simulink model "TEST"  (R2021a)
settings: Solver=VariableStepAuto  StartTime=0.0  StopTime=50  FixedStep=0.001  RelTol=1e-3
values from neighbouring files (symbols this model uses):
  B = inv(N)    [Para.m]    (also in Parameters.m = inv(N)*[zeros(3);eye(3)])
  dtheta_LMO = sqrt(muy/r_LMO^3)    [Para.m]    (also in Parameters.m)
  i0_LMO = pi/6    (= 0.523598775598)    [Para.m]    (also in Parameters.m)
  N = [eye(3) zeros(3);zeros(3) J]    [Dynamics.m]    (also in Para.m; Parameters.m)
  Omega0_LMO = pi/9    (= 0.349065850399)    [Para.m]    (also in Parameters.m)
  R = eye(6)    [Para.m]    (also in Parameters.m = eye(3))
  S = [0 0 0 0.5 0 0;           0 0 0 0 0.5 0;           0 0 0 0 0 0.5;           f41 0 0 0 0 f46;           0 f52 0 0 0 0;           0 0 f63 f64 0 0]    [Para.m]    (also in Parameters.m; crossMatrix.m = [0 -q3 q2;           q3 0 -q1;           -q2 q1 0])
  theta0_LMO = pi/3    (= 1.0471975512)    [Para.m]    (also in Parameters.m)
undefined symbols (not defined in the file or in its folder): F
libraries: dspsrcs4 x1
settings Model: Creator=VTX  LastModifiedBy=VTX

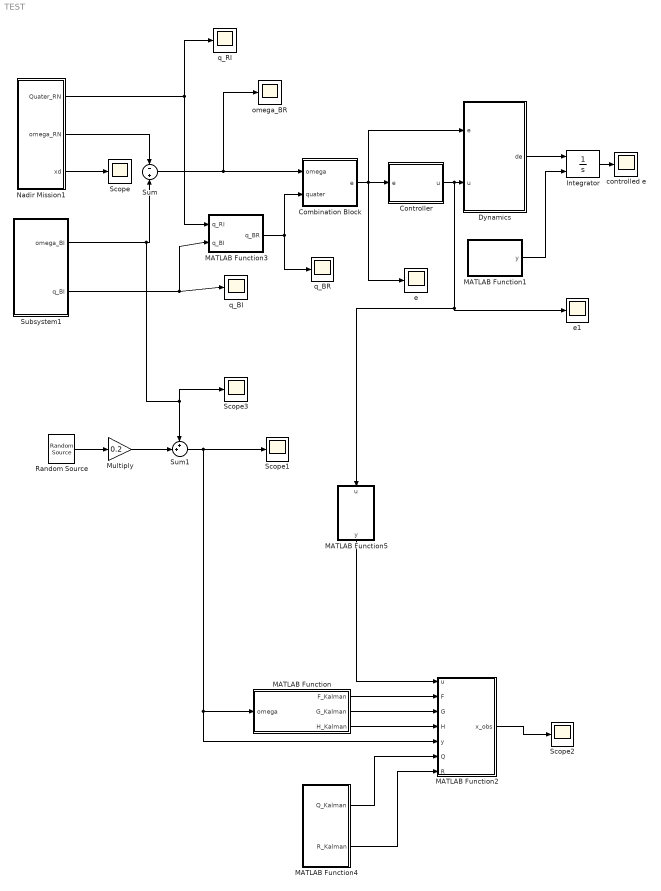
== system TEST ==
  Combination Block : Subsystem
  Controller : MATLAB Function  TreatAsAtomicUnit=on
  Dynamics : MATLAB Function  TreatAsAtomicUnit=on
  Integrator : Integrator  InitialConditionSource=external
  MATLAB Function : MATLAB Function  TreatAsAtomicUnit=on
  MATLAB Function1 : MATLAB Function  TreatAsAtomicUnit=on
  MATLAB Function2 : MATLAB Function  TreatAsAtomicUnit=on
  MATLAB Function3 : MATLAB Function  TreatAsAtomicUnit=on
  MATLAB Function4 : MATLAB Function  TreatAsAtomicUnit=on
  MATLAB Function5 : MATLAB Function  TreatAsAtomicUnit=on
  Multiply : Gain  Gain=0.2
  Nadir Mission1 : Subsystem
  Random Source : dspsrcs4/Random Source  SrcType=Uniform  NormMethod=Ziggurat  CltLength=12  MinVal=0  MaxVal=1  MeanVal=0  VarVal=1  RepMode=Not repeatable  rawSeed=1  IsInherit=off  SampMode=Discrete  SampTime=0.05  SampFrame=1  DataType=Double  OutComplex=Real  OutputFrames=off
  Scope{,1..3} (4 alike) : Scope
  Subsystem1 : Subsystem
  Sum : Sum  Inputs=-|+
  Sum1 : Sum  Inputs=++|
  controlled e : Scope
  e : Scope
  e1 : Scope
  omega_BR : Scope
  q_BI : Scope
  q_BR : Scope
  q_RI : Scope
  wires:
  Controller/1(u) -> MATLAB Function5/1(u), e1/1, Dynamics/2(u)
  Integrator/1 -> controlled e/1
  Dynamics/1(de) -> Integrator/1
  Nadir Mission1/2(omega_RN) -> Sum/1
  Nadir Mission1/3(xd) -> Scope/1
  Nadir Mission1/1(Quater_RN) -> q_RI/1, MATLAB Function3/1(q_RI)
  MATLAB Function3/1(q_BR) -> Combination Block/2(quater), q_BR/1
  Combination Block/1(e) -> e/1, Dynamics/1(e), Controller/1(e)
  Sum/1 -> Combination Block/1(omega), omega_BR/1
  MATLAB Function1/1(y) -> Integrator/2
  Subsystem1/1(omega_BI) -> Scope3/1, Sum1/1, Sum/2
  Subsystem1/2(q_BI) -> q_BI/1, MATLAB Function3/2(q_BI)
  Sum1/1 -> MATLAB Function2/5(y), MATLAB Function/1(omega), Scope1/1
  Random Source/1 -> Multiply/1
  Multiply/1 -> Sum1/2
  MATLAB Function/1(F_Kalman) -> MATLAB Function2/2(F)
  MATLAB Function/2(G_Kalman) -> MATLAB Function2/3(G)
  MATLAB Function/3(H_Kalman) -> MATLAB Function2/4(H)
  MATLAB Function4/1(Q_Kalman) -> MATLAB Function2/6(Q)
  MATLAB Function4/2(R_Kalman) -> MATLAB Function2/7(R)
  MATLAB Function2/1(x_obs) -> Scope2/1
  MATLAB Function5/1(y) -> MATLAB Function2/1(u)

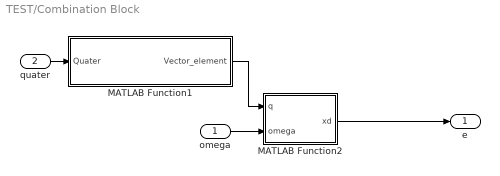
== system TEST/Combination Block ==
  omega : Inport
  quater : Inport  Port=2
  MATLAB Function1 : MATLAB Function  TreatAsAtomicUnit=on
  MATLAB Function2 : MATLAB Function  TreatAsAtomicUnit=on
  e : Outport
  wires:
  MATLAB Function2/1(xd) -> e/1
  MATLAB Function1/1(Vector_element) -> MATLAB Function2/1(q)
  quater/1 -> MATLAB Function1/1(Quater)
  omega/1 -> MATLAB Function2/2(omega)

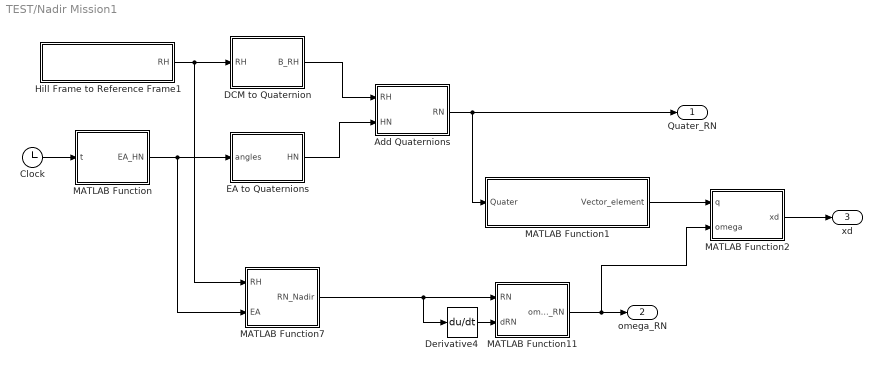
== system TEST/Nadir Mission1 ==
  Add Quaternions : MATLAB Function  TreatAsAtomicUnit=on
  Clock : Clock
  DCM to Quaternion : MATLAB Function  TreatAsAtomicUnit=on
  Derivative4 : Derivative
  EA to Quaternions : MATLAB Function  TreatAsAtomicUnit=on
  Hill Frame to Reference Frame1 : MATLAB Function  TreatAsAtomicUnit=on
  MATLAB Function : MATLAB Function  TreatAsAtomicUnit=on
  MATLAB Function1 : MATLAB Function  TreatAsAtomicUnit=on
  MATLAB Function11 : MATLAB Function  TreatAsAtomicUnit=on
  MATLAB Function2 : MATLAB Function  TreatAsAtomicUnit=on
  MATLAB Function7 : MATLAB Function  TreatAsAtomicUnit=on
  Quater_RN : Outport
  omega_RN : Outport  Port=2
  xd : Outport  Port=3
  wires:
  Hill Frame to Reference Frame1/1(RH) -> MATLAB Function7/1(RH), DCM to Quaternion/1(RH)
  MATLAB Function/1(EA_HN) -> MATLAB Function7/2(EA), EA to Quaternions/1(angles)
  Clock/1 -> MATLAB Function/1(t)
  DCM to Quaternion/1(B_RH) -> Add Quaternions/1(RH)
  EA to Quaternions/1(HN) -> Add Quaternions/2(HN)
  Add Quaternions/1(RN) -> MATLAB Function1/1(Quater), Quater_RN/1
  MATLAB Function7/1(RN_Nadir) -> Derivative4/1, MATLAB Function11/1(RN)
  Derivative4/1 -> MATLAB Function11/2(dRN)
  MATLAB Function11/1(omega_RN) -> MATLAB Function2/2(omega), omega_RN/1
  MATLAB Function1/1(Vector_element) -> MATLAB Function2/1(q)
  MATLAB Function2/1(xd) -> xd/1

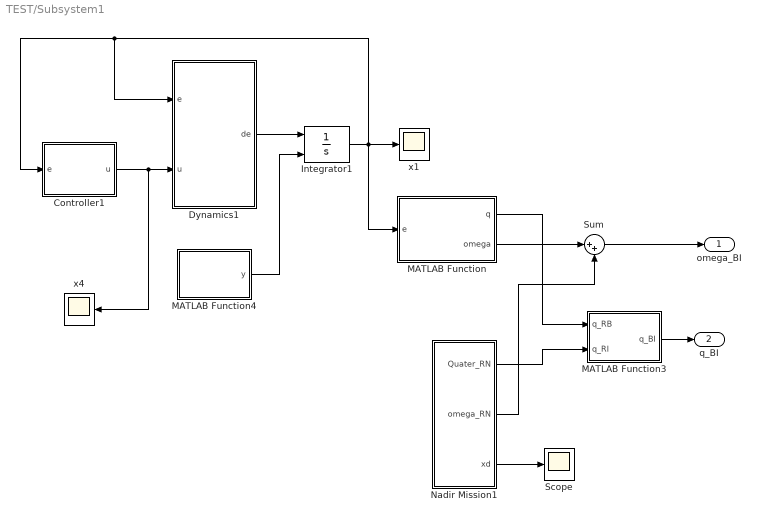
== system TEST/Subsystem1 ==
  Controller1 : MATLAB Function  TreatAsAtomicUnit=on
  Dynamics1 : MATLAB Function  TreatAsAtomicUnit=on
  Integrator1 : Integrator  InitialConditionSource=external
  MATLAB Function : MATLAB Function  TreatAsAtomicUnit=on
  MATLAB Function3 : MATLAB Function  TreatAsAtomicUnit=on
  MATLAB Function4 : MATLAB Function  TreatAsAtomicUnit=on
  Nadir Mission1 : Subsystem
  Scope : Scope
  Sum : Sum  Inputs=|++
  x1 : Scope
  x4 : Scope
  omega_BI : Outport
  q_BI : Outport  Port=2
  wires:
  Integrator1/1 -> MATLAB Function/1(e), Dynamics1/1(e), Controller1/1(e), x1/1
  Controller1/1(u) -> x4/1, Dynamics1/2(u)
  Dynamics1/1(de) -> Integrator1/1
  MATLAB Function4/1(y) -> Integrator1/2
  MATLAB Function/2(omega) -> Sum/1
  MATLAB Function/1(q) -> MATLAB Function3/1(q_RB)
  Nadir Mission1/1(Quater_RN) -> MATLAB Function3/2(q_RI)
  Nadir Mission1/2(omega_RN) -> Sum/2
  Nadir Mission1/3(xd) -> Scope/1
  Sum/1 -> omega_BI/1
  MATLAB Function3/1(q_BI) -> q_BI/1

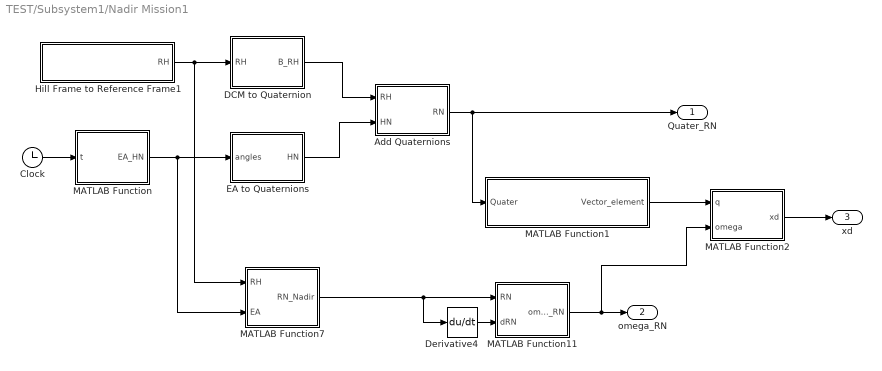
== system TEST/Subsystem1/Nadir Mission1 ==
  Add Quaternions : MATLAB Function  TreatAsAtomicUnit=on
  Clock : Clock
  DCM to Quaternion : MATLAB Function  TreatAsAtomicUnit=on
  Derivative4 : Derivative
  EA to Quaternions : MATLAB Function  TreatAsAtomicUnit=on
  Hill Frame to Reference Frame1 : MATLAB Function  TreatAsAtomicUnit=on
  MATLAB Function : MATLAB Function  TreatAsAtomicUnit=on
  MATLAB Function1 : MATLAB Function  TreatAsAtomicUnit=on
  MATLAB Function11 : MATLAB Function  TreatAsAtomicUnit=on
  MATLAB Function2 : MATLAB Function  TreatAsAtomicUnit=on
  MATLAB Function7 : MATLAB Function  TreatAsAtomicUnit=on
  Quater_RN : Outport
  omega_RN : Outport  Port=2
  xd : Outport  Port=3
  wires:
  Hill Frame to Reference Frame1/1(RH) -> MATLAB Function7/1(RH), DCM to Quaternion/1(RH)
  MATLAB Function/1(EA_HN) -> MATLAB Function7/2(EA), EA to Quaternions/1(angles)
  Clock/1 -> MATLAB Function/1(t)
  DCM to Quaternion/1(B_RH) -> Add Quaternions/1(RH)
  EA to Quaternions/1(HN) -> Add Quaternions/2(HN)
  Add Quaternions/1(RN) -> MATLAB Function1/1(Quater), Quater_RN/1
  MATLAB Function7/1(RN_Nadir) -> Derivative4/1, MATLAB Function11/1(RN)
  Derivative4/1 -> MATLAB Function11/2(dRN)
  MATLAB Function11/1(omega_RN) -> MATLAB Function2/2(omega), omega_RN/1
  MATLAB Function1/1(Vector_element) -> MATLAB Function2/1(q)
  MATLAB Function2/1(xd) -> xd/1

== matlab function TEST/Nadir Mission1/EA to Quaternions ==
  data: angles input; HN output
function HN = EulerAngles313_2_Quaternions(angles)
    Omega = angles(1);
    i = angles(2);
    omega = angles(3);

    q0 = cos(omega/2)*cos(i/2)*cos(Omega/2) - sin(omega/2)*cos(i/2)*sin(Omega/2);
    q1 = cos(omega/2)*sin(i/2)*cos(Omega/2) + sin(omega/2)*sin(i/2)*sin(Omega/2);
    q2 = -sin(omega/2)*sin(i/2)*cos(Omega/2) + cos(omega/2)*sin(i/2)*sin(Omega/2);
    q3 = sin(omega/2)*cos(i/2)*cos(Omega/2) + cos(omega/2)*cos(i/2)*sin(Omega/2);
    
    HN = [q0 q1 q2 q3]';
end

== matlab function TEST/Nadir Mission1/Hill Frame to Reference Frame1 ==
  data: RH output
function RH = fcn()
RH = [-1 0 0;0 1 0;0 0 -1];
end

== matlab function TEST/Nadir Mission1/MATLAB Function ==
  data: t input; EA_HN output; Omega0_LMO parameter; i0_LMO parameter; theta0_LMO parameter; dtheta_LMO parameter
function EA_HN = fcn(t,Omega0_LMO, i0_LMO, theta0_LMO, dtheta_LMO)
    EA_HN = [Omega0_LMO i0_LMO (theta0_LMO + dtheta_LMO*t)]';
end

== matlab function TEST/Nadir Mission1/MATLAB Function11 ==
  data: RN input; omega_RN output; dRN input
function omega_RN = fcn(RN,dRN)
    omega_RN_tidle = -dRN*RN';
    o1 = omega_RN_tidle(3,2);
    o2 = omega_RN_tidle(1,3);
    o3 = omega_RN_tidle(2,1);
    omega_RN = [o1 o2 o3]';
end

== matlab function TEST/Nadir Mission1/MATLAB Function7 ==
  data: RN_Nadir output; RH input; EA input
function RN_Nadir  = fcn(RH,EA)
    Omega = EA(1);
    i = EA(2);
    theta = EA(3);

    %% Rotate about z axis
    Cz1 = [cos(Omega) sin(Omega) 0;-sin(Omega) cos(Omega) 0;0 0 1];

    %% Rotate about x axis
    Cx2 = [1 0 0;0 cos(i) sin(i);0 -sin(i) cos(i)];
    
    %% Rotate about z axis
    Cz3 = [cos(theta) sin(theta) 0;-sin(theta) cos(theta) 0;0 0 1];

    %% DCM from Inertial Frame to Hill Frame
    HN = Cz3*Cx2*Cz1;
    
    %% DCm from Inertial Frame to Reference Frame
    RN_Nadir = RH*HN;
end

== matlab function TEST/Nadir Mission1/MATLAB Function1 ==
  data: Quater input; Vector_element output
function Vector_element = fcn(Quater)
    Vector_element = Quater(2:4);
end

== matlab function TEST/Nadir Mission1/MATLAB Function2 ==
  data: q input; xd output; omega input
function xd = fcn(q,omega)
    xd = [q;omega]; 
end

== matlab function TEST/Controller ==
  data: e input; u output; F parameter; B parameter; R parameter
function u = fcn(e, F, B, R)
%% Controller
   u = -inv(R)*B'*F*e;
end

== matlab function TEST/Combination Block/MATLAB Function1 ==
  data: Quater input; Vector_element output
function Vector_element = fcn(Quater)
    Vector_element = Quater(2:4);
end

== matlab function TEST/Combination Block/MATLAB Function2 ==
  data: q input; xd output; omega input
function xd = fcn(q,omega)
    xd = [q;omega]; 
end

== matlab function TEST/Subsystem1/Controller1 ==
  data: e input; u output; F parameter; B parameter; R parameter
function u = fcn(e, F, B, R)
%% Controller
   u = -inv(R)*B'*F*e;
end

== matlab function TEST/Subsystem1/Dynamics1 ==
  data: e input; de output; u input; N parameter; S parameter
function de  = fcn(e,u,N,S)
%% Quaternions
    %q = [q1 q2 q3]';
    %quater = [q0 q']';

%% State Model: dx = Ax + Bu
    %dx = inv(N)*(S*[q' omega_BR']' + [0 0 0 u']');
    %de = inv(N)*(S*e + [0 0 0 u']');
    de = inv(N)*(S*e + u);
end

== matlab function TEST/MATLAB Function1 ==
  data: y output
function y = fcn()
    y = [0.380636677657970 0.805066318975925 0.0572178012633585 -0.0174532925199433 -0.0305432619099008 0.0383972435438753]';
end

== matlab function TEST/Subsystem1/MATLAB Function ==
  data: e input; q output; omega output
function [q,omega] = fcn(e)
    q_vector = e(1:3);
    omega = e(4:6);
    
    q0 = abs(sqrt(1 - norm(q_vector)^2));
    q = [q0;q_vector];
end

== matlab function TEST/Subsystem1/Nadir Mission1/Add Quaternions ==
  data: RH input; RN output; HN input
function RN = f(RH,HN)
    %% [BN] = [BR]*[RN]
    q0 = RH(1);
    q1 = RH(2);
    q2 = RH(3);
    q3 = RH(4);
    
    Matrix = [q0 -q1 -q2 -q3; ...
              q1 q0 q3 -q2; ...
              q2 -q3 q0 q1; ...
              q3 q2 -q1 q0];
    RN = Matrix*HN;
end

== matlab function TEST/Subsystem1/Nadir Mission1/DCM to Quaternion ==
  data: RH input; B_RH output size=4
function B_RH = fcn(RH)
    trace = RH(1,1) + RH(2,2) + RH(3,3);
    beta0 = (0.25*(1 + trace));
    beta1 = (0.25*(1 + 2*RH(1,1) - trace));
    beta2 = (0.25*(1 + 2*RH(2,2) - trace));
    beta3 = (0.25*(1 + 2*RH(3,3) - trace));
    
    m = max([beta0 beta1 beta2 beta3]);

    B0 = 0; B1 = 0; B2 = 0; B3 = 0;
    
    if beta0 == m
        B0 = sqrt(beta0);
        B1 = (RH(2,3)-RH(3,2))/(4*B0);
        B2 = (RH(3,1)-RH(1,3))/(4*B0);
        B3 = (RH(1,2)-RH(2,1))/(4*B0);
    elseif beta1 == m
        B1 = sqrt(beta1);
        B0 = (RH(2,3)-RH(3,2))/(4*B1);
        B2 = (RH(1,2)+RH(2,1))/(4*B1);
        B3 = (RH(3,1)+RH(1,3))/(4*B1);
    elseif beta2 == m
        B2 = sqrt(beta2);
        B0 = (RH(3,1)-RH(1,3))/(4*B2);
        B1 = (RH(1,2)+RH(2,1))/(4*B2);
        B3 = (RH(2,3)+RH(3,2))/(4*B2);
    elseif beta3 == m
        B3 = sqrt(beta3);
        B0 = (RH(1,2)-RH(2,1))/(4*B3);
        B1 = (RH(3,1)+RH(1,3))/(4*B3);
        B2 = (RH(2,3)+RH(3,2))/(4*B3);
    end
    
    B_RH = [B0 B1 B2 B3]';
end

== matlab function TEST/Subsystem1/Nadir Mission1/EA to Quaternions ==
  data: angles input; HN output
function HN = EulerAngles313_2_Quaternions(angles)
    Omega = angles(1);
    i = angles(2);
    omega = angles(3);

    q0 = cos(omega/2)*cos(i/2)*cos(Omega/2) - sin(omega/2)*cos(i/2)*sin(Omega/2);
    q1 = cos(omega/2)*sin(i/2)*cos(Omega/2) + sin(omega/2)*sin(i/2)*sin(Omega/2);
    q2 = -sin(omega/2)*sin(i/2)*cos(Omega/2) + cos(omega/2)*sin(i/2)*sin(Omega/2);
    q3 = sin(omega/2)*cos(i/2)*cos(Omega/2) + cos(omega/2)*cos(i/2)*sin(Omega/2);
    
    HN = [q0 q1 q2 q3]';
end

== matlab function TEST/Subsystem1/Nadir Mission1/Hill Frame to Reference Frame1 ==
  data: RH output
function RH = fcn()
RH = [-1 0 0;0 1 0;0 0 -1];
end

== matlab function TEST/Subsystem1/Nadir Mission1/MATLAB Function ==
  data: t input; EA_HN output; Omega0_LMO parameter; i0_LMO parameter; theta0_LMO parameter; dtheta_LMO parameter
function EA_HN = fcn(t,Omega0_LMO, i0_LMO, theta0_LMO, dtheta_LMO)
    EA_HN = [Omega0_LMO i0_LMO (theta0_LMO + dtheta_LMO*t)]';
end

== matlab function TEST/Subsystem1/Nadir Mission1/MATLAB Function1 ==
  data: Quater input; Vector_element output
function Vector_element = fcn(Quater)
    Vector_element = Quater(2:4);
end

== matlab function TEST/Dynamics ==
  data: e input; de output; u input; N parameter; S parameter
function de  = fcn(e,u,N,S)
%% Quaternions
    %q = [q1 q2 q3]';
    %quater = [q0 q']';

%% State Model: dx = Ax + Bu
    %dx = inv(N)*(S*[q' omega_BR']' + [0 0 0 u']');
    %de = inv(N)*(S*e + [0 0 0 u']');
    de = inv(N)*(S*e + u);
end

== matlab function TEST/Subsystem1/Nadir Mission1/MATLAB Function11 ==
  data: RN input; omega_RN output; dRN input
function omega_RN = fcn(RN,dRN)
    omega_RN_tidle = -dRN*RN';
    o1 = omega_RN_tidle(3,2);
    o2 = omega_RN_tidle(1,3);
    o3 = omega_RN_tidle(2,1);
    omega_RN = [o1 o2 o3]';
end

== matlab function TEST/Subsystem1/Nadir Mission1/MATLAB Function2 ==
  data: q input; xd output; omega input
function xd = fcn(q,omega)
    xd = [q;omega]; 
end

== matlab function TEST/Subsystem1/Nadir Mission1/MATLAB Function7 ==
  data: RN_Nadir output; RH input; EA input
function RN_Nadir  = fcn(RH,EA)
    Omega = EA(1);
    i = EA(2);
    theta = EA(3);

    %% Rotate about z axis
    Cz1 = [cos(Omega) sin(Omega) 0;-sin(Omega) cos(Omega) 0;0 0 1];

    %% Rotate about x axis
    Cx2 = [1 0 0;0 cos(i) sin(i);0 -sin(i) cos(i)];
    
    %% Rotate about z axis
    Cz3 = [cos(theta) sin(theta) 0;-sin(theta) cos(theta) 0;0 0 1];

    %% DCM from Inertial Frame to Hill Frame
    HN = Cz3*Cx2*Cz1;
    
    %% DCm from Inertial Frame to Reference Frame
    RN_Nadir = RH*HN;
end

== matlab function TEST/Subsystem1/MATLAB Function3 ==
  data: q_BI output; q_RB input; q_RI input
function q_BI = fcn(q_RB, q_RI)
    %% [RI]=[RB].[BI]
    B0 = q_RB(1);
    B1 = q_RB(2);
    B2 = q_RB(3);
    B3 = q_RB(4);
    
    Matrix = [B0 -B1 -B2 -B3; ...
              B1 B0 B3 -B2; ...
              B2 -B3 B0 B1; ...
              B3 B2 -B1 B0];
    q_BI = inv(Matrix)*q_RI;
    q_BR = [q_RB(1);-q_RB(2:4)];
end

== matlab function TEST/Subsystem1/MATLAB Function4 ==
  data: y output
function y = fcn()
    y = [0.380636677657970 0.805066318975925 0.0572178012633585 -0.0174532925199433 -0.0305432619099008 0.0383972435438753]';
end

== matlab function TEST/MATLAB Function ==
  data: F_Kalman output; omega input; G_Kalman output; H_Kalman output; I parameter
function [F_Kalman,G_Kalman,H_Kalman] = fcn(omega, I)
    h = zeros(3,1);

    F_Kalman = inv(I)*(-crossMatrix(omega)*I + crossMatrix(I*omega) + crossMatrix(h));
    G_Kalman = inv(I);
    H_Kalman = eye(3);
end

== matlab function TEST/MATLAB Function2 ==
  data: u input; F input; x_obs output; G input; H input; y input; Q input; R input
function x_obs  = fcn(u,F,G,H,y, Q,R)
%     x = zeros(3,1);
%     P = eye(3);
%     %% Prediction
%     x_pre = F*x + G*u;
%     P_pre = F*P*F' + Q;
% 
%     %% Correction
%     K_Kalman = P_pre*H'*inv(H*P_pre*H' + R);
%     x = x_pre + K_Kalman*(y - H*x_pre);

    x = cell(1,10);
    x{1} = zeros(3,1);

    P = cell(1,10);
    P{1} = eye(3);
    
    for j = 2:10
        %% Prediction
        x_p = F*x{j-1} + G*u;
        P_p = F*P{j-1}*F' + Q;
    
        %% Correction
        K_Kalman = P_p*H'*inv(H*P_p*H' + R);
        x{j} = x_p + K_Kalman*(y - H*x_p);
        P{j} = (eye(3) - K_Kalman*H)*P_p;
    end
    x_obs = x{10};
end

== matlab function TEST/MATLAB Function3 ==
  data: q_RI input; q_BR output; q_BI input
function q_BR = fcn(q_RI,q_BI)
    %% [RI]=[RB].[BI]
    B0 = q_BI(1);
    B1 = q_BI(2);
    B2 = q_BI(3);
    B3 = q_BI(4);
    
    Matrix = [B0 -B1 -B2 -B3; ...
              B1 B0 -B3 B2; ...
              B2 B3 B0 -B1; ...
              B3 -B2 B1 B0];
    q_BR = inv(Matrix)*q_RI;
end

== matlab function TEST/MATLAB Function4 ==
  data: Q_Kalman output; R_Kalman output
function [Q_Kalman,R_Kalman] = fcn()
    %% R_Kalman = sigma_gyro^2*eye(3);
    R_Kalman = 1.9*10^(-7)*eye(3);

    %% Q_Kalman = sigma_Q^2*eye(3);
    Q_Kalman = 10^(-9)*eye(3);
end

== matlab function TEST/MATLAB Function5 ==
  data: u input; y output
function y = fcn(u)
    y = u(4:6);
end

== matlab function TEST/Nadir Mission1/Add Quaternions ==
  data: RH input; RN output; HN input
function RN = f(RH,HN)
    %% [BN] = [BR]*[RN]
    q0 = RH(1);
    q1 = RH(2);
    q2 = RH(3);
    q3 = RH(4);
    
    Matrix = [q0 -q1 -q2 -q3; ...
              q1 q0 q3 -q2; ...
              q2 -q3 q0 q1; ...
              q3 q2 -q1 q0];
    RN = Matrix*HN;
end

== matlab function TEST/Nadir Mission1/DCM to Quaternion ==
  data: RH input; B_RH output size=4
function B_RH = fcn(RH)
    trace = RH(1,1) + RH(2,2) + RH(3,3);
    beta0 = (0.25*(1 + trace));
    beta1 = (0.25*(1 + 2*RH(1,1) - trace));
    beta2 = (0.25*(1 + 2*RH(2,2) - trace));
    beta3 = (0.25*(1 + 2*RH(3,3) - trace));
    
    m = max([beta0 beta1 beta2 beta3]);

    B0 = 0; B1 = 0; B2 = 0; B3 = 0;
    
    if beta0 == m
        B0 = sqrt(beta0);
        B1 = (RH(2,3)-RH(3,2))/(4*B0);
        B2 = (RH(3,1)-RH(1,3))/(4*B0);
        B3 = (RH(1,2)-RH(2,1))/(4*B0);
    elseif beta1 == m
        B1 = sqrt(beta1);
        B0 = (RH(2,3)-RH(3,2))/(4*B1);
        B2 = (RH(1,2)+RH(2,1))/(4*B1);
        B3 = (RH(3,1)+RH(1,3))/(4*B1);
    elseif beta2 == m
        B2 = sqrt(beta2);
        B0 = (RH(3,1)-RH(1,3))/(4*B2);
        B1 = (RH(1,2)+RH(2,1))/(4*B2);
        B3 = (RH(2,3)+RH(3,2))/(4*B2);
    elseif beta3 == m
        B3 = sqrt(beta3);
        B0 = (RH(1,2)-RH(2,1))/(4*B3);
        B1 = (RH(3,1)+RH(1,3))/(4*B3);
        B2 = (RH(2,3)+RH(3,2))/(4*B3);
    end
    
    B_RH = [B0 B1 B2 B3]';
end
